simulink model "part3_3"  (R2018b)
settings: Solver=VariableStepAuto  StartTime=0.0  StopTime=10.0  RelTol=1e-3
libraries: simulink x1
settings Model: Creator=lisazaher  LastModifiedBy=lisazaher

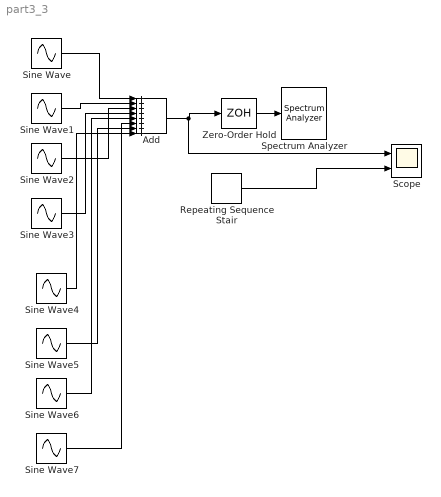
== system part3_3 ==
  Add : Sum  Inputs=++++++++
  Repeating Sequence Stair : simulink/Sources/Repeating Sequence Stair  OutValues=[-1 1].'  tsamp=1/64  OutMin=[]  OutMax=[]  OutDataTypeStr=double  OutputDataTypeScalingMode=double  OutDataType=fixdt(0,8)  ConRadixGroup=Best Precision: Vector-wise  OutScaling=2^-12
  Scope : Scope  NumInputPorts=2
  Sine Wave : Sin  Amplitude=4/pi  Frequency=64*pi  SampleTime=0
  Sine Wave1 : Sin  Amplitude=4/(3*pi)  Frequency=6*32*pi  SampleTime=0
  Sine Wave2 : Sin  Amplitude=4/(5*pi)  Frequency=10*pi*32  SampleTime=0
  Sine Wave3 : Sin  Amplitude=4/(7*pi)  Frequency=14*pi*32  SampleTime=0
  Sine Wave4 : Sin  Amplitude=4/(9*pi)  Frequency=32*18*pi  SampleTime=0
  Sine Wave5 : Sin  Amplitude=4/(11*pi)  Frequency=22*32*pi  SampleTime=0
  Sine Wave6 : Sin  Amplitude=4/(13*pi)  Frequency=26*pi*32  SampleTime=0
  Sine Wave7 : Sin  Amplitude=4/(15*pi)  Frequency=30*pi*32  SampleTime=0
  Spectrum Analyzer : SpectrumAnalyzer
  Zero-Order Hold : ZeroOrderHold  SampleTime=2^-10
  wires:
  Add/1 -> Scope/1, Zero-Order Hold/1
  Sine Wave1/1 -> Add/2
  Sine Wave3/1 -> Add/4
  Sine Wave/1 -> Add/1
  Sine Wave2/1 -> Add/3
  Repeating Sequence Stair/1 -> Scope/2
  Zero-Order Hold/1 -> Spectrum Analyzer/1
  Sine Wave4/1 -> Add/8
  Sine Wave5/1 -> Add/7
  Sine Wave6/1 -> Add/5
  Sine Wave7/1 -> Add/6
